simulink model "VFlexP"  (R2025a)
settings: Solver=ode23tb  StartTime=0.0  StopTime=40  FixedStep=5e-5
model workspace (MAT data in the model file):
  DCop_DCBUCK : object (value not decoded)
  Grid_CCVSC_idx = [2; 3; 4; 5; 6; 7; 8; 9; 10; 11; 12]
  Grid_CCVSCs = 1
  Grid_CCVSCs_buses = 1
  Grid_CCVSCs_toM = [0 1 0 0 0 0 0 0 0 0 0 0 ... (781 elements, 71x11)]
  Grid_C_Lines = [0.1 0.1 0.1 0.1]
  Grid_Cbuses = [0.05000002 0.10000002 0.10000002 0.10000002 0.05000002]
  Grid_DC : object (value not decoded)
  Grid_DCop_DCBUCK : object (value not decoded)
  Grid_DCop_DC_PES : object (value not decoded)
  Grid_DFIGs = 1
  Grid_DFIGs_buses = 1
  Grid_DGs : string (value not decoded)
  Grid_From_buses = [1 2 4 4]
  Grid_GFls = 1
  Grid_GFls_buses = 1
  Grid_GFr_idx = [1; 2; 3]
  Grid_GFrs = 1
  Grid_GFrs_buses = 1
  Grid_GFrs_toM = [1 0 0 0 0 0 0 0 0 1 0 0 ... (15 elements, 5x3)]
  Grid_IG_idx = 1
  Grid_IGs = 1
  Grid_IGs_buses = 1
  Grid_IGs_toM = [1; 0]
  Grid_L_Lines = [0.5 0.5 0.5 0.5]
  Grid_L_Loads = [0.000959999944704 0.000156249997559 0.00154855477548]
  Grid_Lines_fromM : object (value not decoded)
  Grid_Lines_toM : object (value not decoded)
  Grid_Load_buses = [2; 3; 4]
  Grid_Load_busesDC = []
  Grid_MGES_idx = [1; 2; 3]
  Grid_MGESs = 1
  Grid_MGESs_buses = [1; 5; 3]
  Grid_MGESs_toM = [1 0 0 0 0 0 0 0 0 1 0 0 ... (15 elements, 5x3)]
  Grid_MSGs = 1
  Grid_MSGs_buses = 1
  Grid_Nbuses = 5
  Grid_PQ_gen = [3; 2; 2]
  Grid_Ploads = [1250 4000 1250]
  Grid_PloadsDC = []
  Grid_Ps_lf = [0.274439537683 0.78 0.3]
  Grid_Qloads = [0.3 0.5 0.5]
  Grid_Qs_lf = [-0.0366071562958 0.126505596722 -0.0162964024532]
  Grid_R_Lines = [0.01 0.01 0.01 0.01]
  Grid_R_Loads = [3.9999997696 1.24999998047 3.8713869387]
  Grid_R_Loads_DC = 0
  Grid_Rcf = [50000000 50000000 50000000 50000000 50000000]
  Grid_SCs = 1
  Grid_SCs_buses = 1
  Grid_SG_idx = 1
  Grid_SGs = 1
  Grid_SGs_buses = 1
  Grid_SGs_toM = [1; 0]
  Grid_To_buses = [2 3 3 5]
  Grid_VCVSC_idx = [1; 2; 3; 4; 5; 6; 7; 8; 9; 10; 11; 12]
  Grid_VCVSCs = 1
  Grid_VCVSCs_buses = [1; 2; 3; 6; 8; 9; 12; 58; 59; 60; 63; 65]
  Grid_VCVSCs_toM = [1 0 0 0 0 0 0 0 0 0 0 0 ... (852 elements, 71x12)]
  Grid_VSM_idx = [1; 2; 3]
  Grid_VSMs = 1
  Grid_VSMs_buses = 1
  Grid_VSMs_toM = [1 0 0 0 0 0 0 0 0 1 0 0 ... (15 elements, 5x3)]
  Grid_admitt_matrix = [2.15353135314-19.7953135314i  -1.9801980198+19.801980198i; -1.9801980198+19.801980198i  2.15353135314-19.7953135314i]
  Grid_admitt_matrix_noloads = [1.98686468647-19.7953135314i  -1.9801980198+19.801980198i; -1.9801980198+19.801980198i  1.98686468647-19.7953135314i]
  Grid_bus = [1; 2; 6; 7; 8]
  Grid_busDC_complexity = [1 1 1]
  Grid_busDC_complexity_PF = [2 2 2]
  Grid_bus_complexity = [1 1 1 1 1]
  Grid_bus_complexity_PF = [1 1 1 1 1]
  Grid_buses_lf = [1; 5; 3]
  Grid_conductance_matrix = [100.00000002  -100  0; -100  200.00000002  -100; 0  -100  100.00000002]
  Grid_conductance_matrix_noloads = [100.00000002  -100  0; -100  200.00000002  -100; 0  -100  100.00000002]
  Grid_fref : object (value not decoded)
  Grid_gen_static_params : mBase (value not decoded)
  Grid_iPs_lf = [3.64378984326 1.28205128205 3.33333333333]
  Grid_iQs_lf = [-27.3170631425 7.90478860943 -61.3632366329]
  Grid_iadmitt_matrix = [2.88165849328-0.0982918688642i  2.87905051706-0.123273862303i; 2.87905051706-0.123273862303i  2.88165849328-0.0982918688642i]
  Grid_iadmitt_matrix_noloads = [37.5012524798-37.4874983544i  37.4987475202-37.5125016456i; 37.4987475202-37.5125016456i  37.5012524798-37.4874983544i]
  Grid_iconductance_matrix = [16666671.4556  16666671.4489  16666671.4456; 16666671.4489  16666671.4522  16666671.4489; 16666671.4456  16666671.4489  16666671.4556]
  Grid_iconductance_matrix_noloads = [16666671.4556  16666671.4489  16666671.4456; 16666671.4489  16666671.4522  16666671.4489; 16666671.4456  16666671.4489  16666671.4556]
  Grid_init_OK_bool = 1
  Grid_intconv_PF : object (value not decoded)
  Grid_lf_op : op_report (value not decoded)
  Grid_lineDC_complexity = [1 1]
  Grid_lineDC_complexity_PF = [2 2]
  Grid_line_complexity = [1 1 1 1]
  Grid_line_complexity_PF = [3 3 3 3]
  Grid_loadDC_complexity = []
  Grid_loadDC_complexity_PF = []
  Grid_load_complexity = [3 3 3]
  Grid_load_complexity_PF = [4 4 4]
  Grid_opDC_CCVSC : object (value not decoded)
  Grid_opDC_VSM : object (value not decoded)
  Grid_opGFr : object (value not decoded)
  Grid_opVCVSC : object (value not decoded)
  Grid_op_CCVSC : object (value not decoded)
  Grid_op_IG : object (value not decoded)
  Grid_op_MGES : object (value not decoded)
  Grid_op_SG : object (value not decoded)
  Grid_op_VSM : object (value not decoded)
  Grid_shift_lines = [0 0 0 0]
  Grid_tap_lines = [1 1 1 1]
  Grid_v_buses_mod = [1 1 1 0.9837920967 1]
  LinsysParamChangeStruct : Param1 (value not decoded)
  Lline = 0.01
  Rline = 1e-05
  linsys : object (value not decoded)
symbols that are objects in the model workspace (value not decoded): Grid_DCop_DC_PES, Grid_DCop_DCBUCK, Grid_op_CCVSC, Grid_op_IG, Grid_op_MGES, Grid_op_SG, Grid_op_VSM, Grid_opDC_CCVSC, Grid_opDC_VSM, Grid_opGFr, Grid_opVCVSC
undefined symbols (not defined in the file): block_buses_DC, block_idx, CCVSC_idx, Cf, costs, costs2, D, DFIGs_nodes, DiscIntNeverNeededParam, entity, Fb, Fi, From_nodes, grid_linsys, Grid_op_DFIG, Grid_op_DFIG_PQ, Grid_op_MSG, Grid_op_SC, Grid_op_VCVSC, H, initial_states_grid, K_1, K_3, K_5, K_A, K_C, K_IM, K_IR, K_P, K_PM, K_PR, K_S1, K_S2, K_S3, Ki_w, Kic, Kiv, Kp_id, Kp_theta, Kp_w, Kpc, Kpv, last_send, Lc, Lf, Lfd, Lkd1, Lkd2, Lkq1, Lkq2, Lkq3, Lmd, Lmq, Lsd, Lsq, m, M, Matrix_flux_to_i, mp, MSGs_buses ... (+44)
libraries: simulink x1048, eeGeneralControl x12
(part 27 of 50)

== system VFlexP/Grid/Generators/DFIG/GSC Control/PI Estator Current d ==
  in : Inport
  Gain : Gain  Gain=Kp_ia
  Gain1 : Gain  Gain=Ki_ia
  Sum : Sum  Inputs=++|
  xa2 : Integrator  InitialCondition=Grid_op_DFIG.op.States(4).x'
  out : Outport  VectorParamsAs1DForOutWhenUnconnected=off
  wires:
  xa2/1 -> Sum/2
  Gain/1 -> Sum/1
  in/1 -> Gain1/1, Gain/1
  Sum/1 -> out/1
  Gain1/1 -> xa2/1

== system VFlexP/Grid/Generators/DFIG/GSC Control/PI Estator Current q ==
  in : Inport
  Gain : Gain  Gain=Kp_ia
  Gain1 : Gain  Gain=Ki_ia
  Sum : Sum  Inputs=++|
  xa1 : Integrator  InitialCondition=Grid_op_DFIG.op.States(5).x'
  out : Outport  VectorParamsAs1DForOutWhenUnconnected=off
  wires:
  Gain1/1 -> xa1/1
  Sum/1 -> out/1
  in/1 -> Gain/1, Gain1/1
  Gain/1 -> Sum/1
  xa1/1 -> Sum/2

== system VFlexP/Grid/Generators/DFIG/GSC Control/Subsystem1 ==
  ws : Inport
  vaq' : Inport  Port=2
  vsq : Inport  Port=3
  iad : Inport  Port=4
  Gain1 : Gain  Gain=La_pu
  Product1 : Product
  Sum4 : Sum  Inputs=-|+|-  InputSameDT=on  SaturateOnIntegerOverflow=on  OutDataTypeStr=Inherit: Same as first input
  vadq : Outport
  wires:
  iad/1 -> Product1/2
  Gain1/1 -> Product1/1
  vaq'/1 -> Sum4/1
  Sum4/1 -> vadq/1  "vadq"
  Product1/1 -> Sum4/3
  ws/1 -> Gain1/1
  vsq/1 -> Sum4/2

== system VFlexP/Grid/Generators/DFIG/GSC Control/Subsystem3 ==
  vad' : Inport
  vd : Inport  Port=2
  iaq : Inport  Port=3
  ws : Inport  Port=4
  Gain1 : Gain  Gain=La_pu
  Product1 : Product
  Sum4 : Sum  Inputs=-|+|+  InputSameDT=on  SaturateOnIntegerOverflow=on  OutDataTypeStr=Inherit: Same as first input
  vad : Outport
  wires:
  iaq/1 -> Product1/2
  ws/1 -> Gain1/1
  Product1/1 -> Sum4/3
  Sum4/1 -> vad/1  "vadq"
  vd/1 -> Sum4/2
  vad'/1 -> Sum4/1
  Gain1/1 -> Product1/1

== system VFlexP/Grid/Generators/DFIG/RSC Control/PI Rotor Current d ==
  in : Inport
  Gain : Gain  Gain=Kp_ir
  Gain1 : Gain  Gain=Ki_ir
  Sum : Sum  Inputs=++|
  xr1 : Integrator  InitialCondition=Grid_op_DFIG.op.States(12).x'
  out : Outport  VectorParamsAs1DForOutWhenUnconnected=off
  wires:
  Gain1/1 -> xr1/1
  Sum/1 -> out/1
  in/1 -> Gain/1, Gain1/1
  Gain/1 -> Sum/1
  xr1/1 -> Sum/2

== system VFlexP/Grid/Generators/DFIG/RSC Control/PI Rotor Current q ==
  in : Inport
  Gain : Gain  Gain=Kp_ir
  Gain1 : Gain  Gain=Ki_ir
  Sum : Sum  Inputs=++|
  xr2 : Integrator  InitialCondition=Grid_op_DFIG.op.States(13).x'
  out : Outport  VectorParamsAs1DForOutWhenUnconnected=off
  wires:
  xr2/1 -> Sum/2
  Gain/1 -> Sum/1
  in/1 -> Gain1/1, Gain/1
  Sum/1 -> out/1
  Gain1/1 -> xr2/1

== system VFlexP/Grid/Generators/DFIG/Slip/PI Slip ==
  in : Inport
  Gain : Gain  Gain=Kp_s
  Gain1 : Gain  Gain=Ki_s
  Sum : Sum  Inputs=++|
  xr3 : Integrator  InitialCondition=Grid_op_DFIG_PQ.op.States(16).x'  UpperSaturationLimit=1.01  LowerSaturationLimit=0.99
  out : Outport  VectorParamsAs1DForOutWhenUnconnected=off
  wires:
  xr3/1 -> Sum/2
  Gain/1 -> Sum/1
  in/1 -> Gain1/1, Gain/1
  Sum/1 -> out/1
  Gain1/1 -> xr3/1

== system VFlexP/Grid/Generators/DFIG/Stator circuit/Subsystem1 ==
  vd : Inport
  vq : Inport  Port=2
  id : Inport  Port=3
  iq : Inport  Port=4
  s*ws : Inport  Port=5
  Gain1 : Gain  Gain=Rr_pu
  Gain6 : Gain  Gain=Rr_pu
  Gain7 : Gain  Gain=-1
  Product{1..4} (4 alike) : Product
  Selector8 : Selector  InputPortWidth=length(fref.ref_units)  IndexOptions=Index vector (dialog)  Indices=block_fref  OutputSizes=1
  Sum1 : Sum  Inputs=-|+|-  InputSameDT=on  SaturateOnIntegerOverflow=on  OutDataTypeStr=Inherit: Same as first input
  Sum4 : Sum  Inputs=-|+|-  InputSameDT=on  SaturateOnIntegerOverflow=on  OutDataTypeStr=Inherit: Same as first input
  psis_d : Integrator  InitialCondition=Grid_op_DFIG.op.States(15).x'
  psis_q : Integrator  InitialCondition=Grid_op_DFIG.op.States(16).x'
  d : Outport
  q : Outport  Port=2
  wires:
  Product1/1 -> Sum4/1
  s*ws/1 -> Product1/1, Product2/2
  Gain6/1 -> Sum4/3
  Product3/1 -> psis_q/1
  Sum1/1 -> Product4/1
  psis_d/1 -> Product1/2, d/1
  Sum4/1 -> Product3/2
  Product4/1 -> psis_d/1
  Gain1/1 -> Sum1/1
  Gain7/1 -> Product2/1
  id/1 -> Gain1/1
  Product2/1 -> Sum1/3
  psis_q/1 -> q/1, Gain7/1
  iq/1 -> Gain6/1
  vd/1 -> Sum1/2
  vq/1 -> Sum4/2
  Selector8/1 -> Product3/1, Product4/2
  [omega_base] -> Selector8/1

== system VFlexP/Grid/Generators/DFIG/Stator circuit/Subsystem2 ==
  vad : Inport
  vaq : Inport  Port=2
  id : Inport  Port=3
  iq : Inport  Port=4
  ws : Inport  Port=5
  vsd : Inport  Port=6
  vsq : Inport  Port=7
  Gain1 : Gain  Gain=Ra_pu
  Gain6 : Gain  Gain=Ra_pu
  Gain7 : Gain  Gain=-1
  Product{1..4} (4 alike) : Product
  Selector8 : Selector  InputPortWidth=length(fref.ref_units)  IndexOptions=Index vector (dialog)  Indices=block_fref  OutputSizes=1
  Sum1 : Sum  Inputs=-|+|-|-  InputSameDT=on  SaturateOnIntegerOverflow=on  OutDataTypeStr=Inherit: Same as first input
  Sum2 : Sum  Inputs=-|+|-|-  InputSameDT=on  SaturateOnIntegerOverflow=on  OutDataTypeStr=Inherit: Same as first input
  psis_d : Integrator  InitialCondition=Grid_op_DFIG.op.States(17).x'
  psis_q : Integrator  InitialCondition=Grid_op_DFIG.op.States(18).x'
  d : Outport
  q : Outport  Port=2
  wires:
  iq/1 -> Gain6/1
  psis_q/1 -> Gain7/1, q/1
  Product2/1 -> Sum1/3
  id/1 -> Gain1/1
  Gain7/1 -> Product2/1
  Gain1/1 -> Sum1/1
  Product4/1 -> psis_d/1
  Sum2/1 -> Product3/2
  psis_d/1 -> Product1/2, d/1
  Sum1/1 -> Product4/1
  Product3/1 -> psis_q/1
  ws/1 -> Product2/2, Product1/1
  vsd/1 -> Sum1/2
  vad/1 -> Sum1/4
  Gain6/1 -> Sum2/4
  vsq/1 -> Sum2/2
  Product1/1 -> Sum2/1
  vaq/1 -> Sum2/3
  Selector8/1 -> Product3/1, Product4/2
  [omega_base] -> Selector8/1

== system VFlexP/Grid/Generators/DFIG/Stator circuit/Subsystem3 ==
  vd : Inport
  vq : Inport  Port=2
  id : Inport  Port=3
  iq : Inport  Port=4
  ws : Inport  Port=5
  Gain1 : Gain  Gain=Rs_pu
  Gain6 : Gain  Gain=Rs_pu
  Gain7 : Gain  Gain=-1
  Product{1..4} (4 alike) : Product
  Selector8 : Selector  InputPortWidth=length(fref.ref_units)  IndexOptions=Index vector (dialog)  Indices=block_fref  OutputSizes=1
  Sum1 : Sum  Inputs=-|+|-  InputSameDT=on  SaturateOnIntegerOverflow=on  OutDataTypeStr=Inherit: Same as first input
  Sum4 : Sum  Inputs=-|+|-  InputSameDT=on  SaturateOnIntegerOverflow=on  OutDataTypeStr=Inherit: Same as first input
  psis_d : Integrator  InitialCondition=Grid_op_DFIG.op.States(19).x'
  psis_q : Integrator  InitialCondition=Grid_op_DFIG.op.States(20).x'
  d : Outport
  q : Outport  Port=2
  wires:
  vq/1 -> Sum4/2
  vd/1 -> Sum1/2
  iq/1 -> Gain6/1
  psis_q/1 -> q/1, Gain7/1
  Product2/1 -> Sum1/3
  id/1 -> Gain1/1
  Gain7/1 -> Product2/1
  Product4/1 -> psis_d/1
  Sum4/1 -> Product3/2
  psis_d/1 -> d/1, Product1/2
  Sum1/1 -> Product4/1
  Product3/1 -> psis_q/1
  ws/1 -> Product2/2, Product1/1
  Product1/1 -> Sum4/1
  Gain1/1 -> Sum1/1
  Gain6/1 -> Sum4/3
  Selector8/1 -> Product3/1, Product4/2
  [omega_base] -> Selector8/1

== system VFlexP/Grid/Generators/DFIG/Vc control/PI Vc2 ==
  in : Inport
  Gain : Gain  Gain=Kp_vc2
  Gain1 : Gain  Gain=Ki_vc2
  Sum : Sum  Inputs=++|
  xa3 : Integrator  InitialCondition=Grid_op_DFIG.op.States(22).x'
  out : Outport  VectorParamsAs1DForOutWhenUnconnected=off
  wires:
  Gain1/1 -> xa3/1
  Sum/1 -> out/1
  in/1 -> Gain/1, Gain1/1
  Gain/1 -> Sum/1
  xa3/1 -> Sum/2

== system VFlexP/Grid/Generators/GFl/CC/dynamic ==
  idref : Inport
  iqref : Inport  Port=2
  vod : Inport  Port=3
  voq : Inport  Port=4
  omega : Inport  Port=5
  "Lf " : Gain  Gain=Lf
  Lf1 : Gain  Gain=Lf
  Product : Product
  Product3 : Product
  RL : Subsystem  Variant=on  VariantControlMode=label  LabelModeActiveChoice=dynamic  mask(Line){dynamic=Dynamic, R=Rf, L=Lf}
      mask prompts: dynamic "Dynamic behavior"; R "Series resistance (p.u.)"; L "Inductance (p.u.)"
      mask init: same as VFlexP/Grid/Generators/GFr/RL out
      mask Help: web('Documentation/RL.html')
      mask TypeOptions dynamic: Static | Dynamic | Static omega
  Subsystem : Subsystem
  Subsystem1 : Subsystem
  Sum1 : Sum  Inputs=++|
  Sum2 : Sum  Inputs=++|
  Sum8 : Sum  Inputs=-+|
  Sum9 : Sum  Inputs=|++
  idiref : Outport
  iqiref : Outport  Port=2
  wires:
  RL/2(iq) -> iqiref/1, Subsystem1/2(y), "Lf "/1
  Subsystem1/1(Out1) -> Sum9/1
  [omega] -> Product3/1  "omega"
  "Lf "/1 -> Product/1
  Product3/1 -> Sum9/2
  Lf1/1 -> Product3/2
  [omega] -> Product/2
  Product/1 -> Sum8/1
  iqref/1 -> Subsystem1/1(ref)  "iqref"
  Sum8/1 -> Sum1/2
  Sum9/1 -> Sum2/2
  [vod] -> Sum1/1
  [voq] -> Sum2/1
  omega/1 -> [omega]  "omega"
  voq/1 -> [voq]  "ioq"
  vod/1 -> [vod]  "iod"
  [vod] -> RL/2(v_out_d)
  [voq] -> RL/4(v_out_q)
  Sum1/1 -> RL/1(v_in_d)
  Sum2/1 -> RL/3(v_in_q)
  RL/1(id) -> Subsystem/2(y), Lf1/1, idiref/1
  idref/1 -> Subsystem/1(ref)  "idref"
  Subsystem/1(Out1) -> Sum8/2
  [omega] -> RL/5(omega)

== system VFlexP/Grid/Generators/GFl/CC/static ==
  idref : Inport
  iqref : Inport  Port=2
  vod : Inport  Port=3
  voq : Inport  Port=4
  omega : Inport  Port=5
  Terminator : Terminator
  Terminator1 : Terminator
  Terminator2 : Terminator
  idiref : Outport
  iqiref : Outport  Port=2
  wires:
  voq/1 -> Terminator1/1  "voq"
  vod/1 -> Terminator/1  "vod"
  idref/1 -> idiref/1  "idref"
  iqref/1 -> iqiref/1  "iqref"
  omega/1 -> Terminator2/1  "omega"

== system VFlexP/Grid/Generators/GFl/PC/LPF_d ==
  In1 : Inport
  Gain : Gain  Gain=iTf
  I : Integrator  InitialCondition=Grid_op_CCVSC.op.States(8).x'
  Sum4 : Sum  Inputs=|+-
  Out1 : Outport
  wires:
  Gain/1 -> I/1
  Sum4/1 -> Gain/1
  In1/1 -> Sum4/1
  I/1 -> Sum4/2, Out1/1

== system VFlexP/Grid/Generators/GFl/PC/LPF_q ==
  In1 : Inport
  Gain : Gain  Gain=iTf
  I : Integrator  InitialCondition=Grid_op_CCVSC.op.States(9).x'
  Sum4 : Sum  Inputs=|+-
  Out1 : Outport
  wires:
  Gain/1 -> I/1
  I/1 -> Sum4/2, Out1/1
  In1/1 -> Sum4/1
  Sum4/1 -> Gain/1

== system VFlexP/Grid/Generators/GFl/PC/Saturation ==
  ildref : Inport
  ilqref : Inport  Port=2
  Abs : Abs  ZeroCross=off  SaturateOnIntegerOverflow=off
  Abs1 : Abs  ZeroCross=off  SaturateOnIntegerOverflow=off
  Abs2 : Abs  ZeroCross=off  SaturateOnIntegerOverflow=off
  Divide2 : Product  Inputs=*/
  Divide3 : Product  Inputs=*/
  Gain : Gain  Gain=-1
  Gain3 : Gain  Gain=-1
  Real-Imag to Complex : RealImagToComplex
  Saturation Dynamic : simulink/Discontinuities/Saturation Dynamic  OutMin=[]  OutMax=[]  OutDataTypeStr=Inherit: Same as second input  OutDataType=fixdt(1, 16)  OutScaling=2^-10  DoSatur=off
  Saturation Dynamic1 : simulink/Discontinuities/Saturation Dynamic  OutMin=[]  OutMax=[]  OutDataTypeStr=Inherit: Same as second input  OutDataType=fixdt(1, 16)  OutScaling=2^-10  DoSatur=off
  y : Outport
  y1 : Outport  Port=2
  wires:
  Gain/1 -> Saturation Dynamic1/3
  Divide3/1 -> Gain/1, Saturation Dynamic1/1
  Divide2/1 -> Gain3/1, Saturation Dynamic/1
  Saturation Dynamic/1 -> y/1
  Abs/1 -> Divide3/2, Divide2/2
  Gain3/1 -> Saturation Dynamic/3
  Abs1/1 -> Divide3/1
  Real-Imag to Complex/1 -> Abs/1
  ilqref/1 -> Abs1/1, Saturation Dynamic1/2, Real-Imag to Complex/2
  Abs2/1 -> Divide2/1
  ildref/1 -> Abs2/1, Saturation Dynamic/2, Real-Imag to Complex/1
  Saturation Dynamic1/1 -> y1/1

== system VFlexP/Grid/Generators/GFl/PLL/dynamic ==
  vq : Inport
  omega : Inport  Port=2
  voutangle : Inport  Port=3
  PLL : Subsystem
  Product : Product
  Selector8 : Selector  InputPortWidth=length(fref.ref_units)  IndexOptions=Index vector (dialog)  Indices=block_fref  OutputSizes=1
  Sum2 : Sum  Inputs=|-+
  Sum3 : Sum  Inputs=+-|
  Terminator : Terminator
  Zero : Constant  Value=0  OutDataTypeStr=Inherit: Inherit via back propagation
  frame : Integrator  InitialCondition=Grid_op_CCVSC.op.States(7).x'  UpperSaturationLimit=pi  LowerSaturationLimit=-pi
  theta : Outport
  omega_point : Outport  Port=2
  wires:
  voutangle/1 -> Terminator/1
  vq/1 -> Sum2/2  "vq"
  omega/1 -> Sum3/2  "omega"
  Zero/1 -> Sum2/1
  frame/1 -> theta/1  "theta"
  Product/1 -> frame/1
  PLL/1(Input2) -> omega_point/1, Sum3/1  "omega2"
  Sum3/1 -> Product/1
  Sum2/1 -> PLL/1(In1)
  [omega_base] -> Selector8/1
  Selector8/1 -> Product/2

== system VFlexP/Grid/Generators/GFl/PLL/static ==
  vq : Inport
  omega : Inport  Port=2
  voutangle : Inport  Port=3
  Gain : Gain  Gain=-1
  Terminator : Terminator
  Terminator1 : Terminator
  Transport Delay : TransportDelay  DelayTime=1e-6  TransDelayFeedthrough=on
  theta : Outport
  omega_point : Outport  Port=2
  wires:
  Transport Delay/1 -> theta/1
  Gain/1 -> Transport Delay/1
  vq/1 -> Terminator/1  "vq"
  omega/1 -> omega_point/1, Terminator1/1  "vq"
  voutangle/1 -> Gain/1

== system VFlexP/Grid/Generators/GFr/PC/LPF_P ==
  P : Inport
  Gain : Gain  Gain=iTf
  I : Integrator
  Sum4 : Sum  Inputs=|+-
  P_f : Outport
  wires:
  Gain/1 -> I/1
  Sum4/1 -> Gain/1
  P/1 -> Sum4/1
  I/1 -> P_f/1, Sum4/2

== system VFlexP/Grid/Generators/GFr/PC/LPF_Q ==
  Q : Inport
  Gain : Gain  Gain=iTf
  I : Integrator
  Sum4 : Sum  Inputs=|+-
  Q_f : Outport
  wires:
  Gain/1 -> I/1
  Q/1 -> Sum4/1
  I/1 -> Q_f/1, Sum4/2
  Sum4/1 -> Gain/1

== system VFlexP/Grid/Generators/GFr/RL out/dynamic ==
  v_in_d : Inport
  v_out_d : Inport  Port=2
  v_in_q : Inport  Port=3
  v_out_q : Inport  Port=4
  Gain1 : Gain  Gain=L
  Gain2 : Gain  Gain=R
  Gain3 : Gain  Gain=R
  Gain4 : Gain  Gain=L
  Gain5 : Gain  Gain=invL
  Gain7 : Gain  Gain=invL
  Product{,1..3} (4 alike) : Product
  Selector1 : Selector  InputPortWidth=length(fref.ref_units)  IndexOptions=Index vector (dialog)  Indices=block_fref  OutputSizes=1
  Selector7 : Selector  InputPortWidth=length(fref.ref_units)  IndexOptions=Index vector (dialog)  Indices=block_fref  OutputSizes=1
  Sum4 : Sum  Inputs=+-|
  Sum5 : Sum  Inputs=|-+
  Sum6 : Sum  Inputs=|++
  Sum7 : Sum  Inputs=-+|
  Sum8 : Sum  Inputs=|+-
  Sum9 : Sum  Inputs=-+|
  i_d : Integrator  InitialCondition=Grid_opGFr.id_out
  i_q : Integrator  InitialCondition=Grid_opGFr.iq_out
  id : Outport
  iq : Outport  Port=2
  v_outd : Outport  Port=3
  v_outq : Outport  Port=4
  wires:
  v_out_q/1 -> v_outq/1, Sum9/1  "v_out_q"
  v_out_d/1 -> v_outd/1, Sum7/1  "v_out_d"
  Sum9/1 -> Sum8/1
  Gain1/1 -> Product1/2
  i_q/1 -> iq/1, Gain4/1, Gain3/1  "iq"
  Sum5/1 -> Sum9/2
  Gain3/1 -> Sum5/1
  Sum7/1 -> Sum6/1
  Gain4/1 -> Product/1
  Product1/1 -> Sum8/2
  Sum4/1 -> Sum7/2
  Sum8/1 -> Gain7/1
  Product/1 -> Sum6/2
  [omega_ref] -> Selector7/1  "omega"
  Sum6/1 -> Gain5/1
  i_d/1 -> id/1, Gain1/1, Gain2/1  "id"
  Gain2/1 -> Sum4/2
  v_in_d/1 -> Sum4/1  "v_in_d"
  v_in_q/1 -> Sum5/2  "v_in_q"
  Selector7/1 -> Product/2, Product1/1
  Selector1/1 -> Product2/2, Product3/1
  [omega_base] -> Selector1/1
  Product3/1 -> i_q/1
  Gain7/1 -> Product3/2
  Gain5/1 -> Product2/1
  Product2/1 -> i_d/1

== system VFlexP/Grid/Generators/GFr/RL out/static ==
  v_in_d : Inport
  v_out_d : Inport  Port=2
  v_in_q : Inport  Port=3
  v_out_q : Inport  Port=4
  Constant : Constant  Value=R.^2
  Constant1 : Constant
  Divide : Product  Inputs=*/
  Gain : Gain  Gain=L
  Gain1 : Gain  Gain=R
  Gain2 : Gain  Gain=R
  Product{,1..5} (6 alike) : Product
  Selector7 : Selector  InputPortWidth=length(fref.ref_units)  IndexOptions=Index vector (dialog)  Indices=block_fref  OutputSizes=1
  Sum : Sum  Inputs=|++
  Sum1 : Sum  Inputs=|+-
  Sum2 : Sum  Inputs=|+-
  Sum3 : Sum  Inputs=|++
  Sum4 : Sum  Inputs=|-+
  id : Outport
  iq : Outport  Port=2
  v_outd : Outport  Port=3
  v_outq : Outport  Port=4
  wires:
  v_in_d/1 -> Sum1/1  "v_in_d"
  v_out_q/1 -> v_outq/1, Sum2/2  "v_out_q"
  Sum4/1 -> iq/1  "iq"
  Sum3/1 -> id/1  "id"
  Gain1/1 -> Product1/2
  Product2/1 -> Product4/2, Product3/1
  Product4/1 -> Sum4/1
  Divide/1 -> Gain2/1, Gain1/1, Product2/1
  Sum1/1 -> Product1/1, Product4/1  "vd"
  Product3/1 -> Sum3/2
  Constant1/1 -> Divide/1
  Gain/1 -> Product/2, Product/1, Product2/2
  Sum2/1 -> Product5/1, Product3/2  "vq"
  Constant/1 -> Sum/1
  Product5/1 -> Sum4/2
  Product1/1 -> Sum3/1
  Product/1 -> Sum/2
  Gain2/1 -> Product5/2
  Sum/1 -> Divide/2
  v_out_d/1 -> v_outd/1, Sum1/2  "v_out_d"
  v_in_q/1 -> Sum2/1  "v_in_q"
  [omega_ref] -> Selector7/1  "omega"
  Selector7/1 -> Gain/1

== system VFlexP/Grid/Generators/GFr/RL out/static_omega ==
  v_in_d : Inport
  v_out_d : Inport  Port=2
  v_in_q : Inport  Port=3
  v_out_q : Inport  Port=4
  Gain : Gain  Gain=1./(R.^2+L.^2)
  Gain2 : Gain  Gain=1./(R.^2+L.^2)
  Gain3 : Gain  Gain=R
  Gain4 : Gain  Gain=L
  Gain5 : Gain  Gain=L
  Gain6 : Gain  Gain=R
  Sum : Sum  Inputs=|++
  Sum1 : Sum  Inputs=|+-
  Sum2 : Sum  Inputs=|+-
  Sum3 : Sum  Inputs=|-+
  id : Outport
  iq : Outport  Port=2
  v_outd : Outport  Port=3
  v_outq : Outport  Port=4
  wires:
  v_in_q/1 -> Sum2/1  "v_in_q"
  v_in_d/1 -> Sum1/1  "v_in_d"
  v_out_q/1 -> v_outq/1, Sum2/2  "v_out_q"
  v_out_d/1 -> v_outd/1, Sum1/2  "v_out_d"
  Sum1/1 -> Gain/1  "vd"
  Sum2/1 -> Gain2/1  "vq"
  Gain/1 -> Gain5/1, Gain3/1
  Gain3/1 -> Sum/1
  Gain4/1 -> Sum/2
  Gain2/1 -> Gain6/1, Gain4/1
  Sum/1 -> id/1
  Gain5/1 -> Sum3/1
  Sum3/1 -> iq/1
  Gain6/1 -> Sum3/2

== system VFlexP/Grid/Generators/GFr/VCC/dynamic ==
  vodref : Inport
  voqref : Inport  Port=2
  iod : Inport  Port=3
  ioq : Inport  Port=4
  omega : Inport  Port=5
  Cf : Gain  Gain=Cfi
  Cf 1 : Gain  Gain=Cfi
  Constant : Constant  Value=Tint==Inf  VectorParams1D=off
  Constant1 : Constant  Value=Text==Inf  VectorParams1D=off
  Fi : Gain  Gain=Fi
  Fi2 : Gain  Gain=Fi
  "Lf " : Gain  Gain=Lf
  Lf1 : Gain  Gain=Lf
  PIid : Subsystem
  PIiq : Subsystem
  PIvd : Subsystem
  PIvq : Subsystem
  Product{,1..3} (4 alike) : Product
  RC : Subsystem  Variant=on  VariantControlMode=label  LabelModeActiveChoice=dynamic  mask{dynamic=Dynamic, R=Rcf, C=Cfi}
      mask prompts: dynamic "Dynamic behavior"; R "Parallel resistance (p.u.)"; C "Capacitance (p.u.)"
      mask init: same as VFlexP/Grid/DCAC converters/DC_VSM/VCC/dynamic_limiting/RC
      mask TypeOptions dynamic: Dynamic | Static | Static omega
  RL : Subsystem  Variant=on  VariantControlMode=label  LabelModeActiveChoice=dynamic  mask(Line){dynamic=Dynamic, R=Rf, L=Lf}
      mask prompts: dynamic "Dynamic behavior"; R "Series resistance (p.u.)"; L "Inductance (p.u.)"
      mask init: same as VFlexP/Grid/Generators/GFr/RL out
      mask Help: web('Documentation/RL.html')
      mask TypeOptions dynamic: Static | Dynamic | Static omega
  Subsystem : Subsystem
  Subsystem1 : Subsystem
  Sum1 : Sum  Inputs=++|
  Sum2 : Sum  Inputs=-+|
  Sum{3,5..6,9} (4 alike) : Sum  Inputs=|++
  Sum4 : Sum  Inputs=++|
  Sum8 : Sum  Inputs=-+|
  Switch{,1..3} (4 alike) : Switch  Criteria=u2 > Threshold  SaturateOnIntegerOverflow=off  InputSameDT=off
  vidref : Outport
  viqref : Outport  Port=2
  wires:
  Sum5/1 -> Switch1/1, PIiq/1(ref)  "ilqref"
  Product/1 -> Sum8/1
  vodref/1 -> Switch2/1, PIvd/1(ref)  "vodref"
  RC/2(vq) -> PIvq/2(y), Cf/1, Subsystem/4(In4), Sum6/2, Switch3/3  "voq"
  [omega] -> Product/2
  Lf1/1 -> Product3/2
  Fi/1 -> Sum4/1
  voqref/1 -> Switch3/1, PIvq/1(ref)  "voqref"
  Product3/1 -> Sum9/2
  Product2/1 -> Sum3/2
  Cf 1/1 -> Product2/2
  Cf/1 -> Product1/2
  Sum4/1 -> PIid/1(ref), Switch/1  "ildref"
  Product1/1 -> Sum2/1
  iod/1 -> Subsystem1/2(iod), Fi/1  "iod"
  Sum2/1 -> Sum4/2
  "Lf "/1 -> Product/1
  Sum3/1 -> Sum5/1
  [omega] -> Subsystem1/5(In5), Subsystem/5(In5), Product3/1  "omega"
  ioq/1 -> Subsystem1/4(ioq), Fi2/1  "ioq"
  Fi2/1 -> Sum5/2
  PIvd/1(Out1) -> Sum2/2
  PIvq/1(Out1) -> Sum3/1
  PIid/1(Out1) -> Sum8/2
  PIiq/1(Out1) -> Sum9/1
  omega/1 -> Product2/1, [omega]  "omega"
  [omega] -> Product1/1
  RC/1(vd) -> Subsystem/2(In2), Sum1/1, Switch2/3, PIvd/2(y), Cf 1/1
  RL/1(id) -> Switch/3, Lf1/1, PIid/2(y)
  RL/2(iq) -> Switch1/3, PIiq/2(y), "Lf "/1
  Sum8/1 -> Sum1/2  "vidref"
  Sum9/1 -> Sum6/1  "viqref"
  Sum1/1 -> Subsystem/1(In1)
  Sum6/1 -> Subsystem/3(In3)
  Subsystem/1(Out1) -> RL/1(v_in_d)
  Subsystem/2(Out2) -> RL/2(v_out_d)
  Subsystem/3(Out3) -> RL/3(v_in_q)
  Subsystem/4(Out4) -> RL/4(v_out_q)
  Subsystem/5(Out5) -> RL/5(omega)
  Subsystem1/1(Out1) -> RC/1(i_d_in)
  Subsystem1/2(Out2) -> RC/2(i_d_out)
  Subsystem1/3(Out3) -> RC/3(i_q_in)
  Subsystem1/4(Out4) -> RC/4(i_q_out)
  Subsystem1/5(Out5) -> RC/5(omega)
  Switch/1 -> Subsystem1/1(id)
  Switch1/1 -> Subsystem1/3(iq)
  Constant/1 -> Switch1/2, Switch/2
  Switch2/1 -> vidref/1
  Constant1/1 -> Switch3/2, Switch2/2
  Switch3/1 -> viqref/1

== system VFlexP/Grid/Generators/GFr/VCC/dynamic_VC ==
  vodref : Inport
  voqref : Inport  Port=2
  iod : Inport  Port=3
  ioq : Inport  Port=4
  omega : Inport  Port=5
  Cf : Gain  Gain=Cfi
  Cf 1 : Gain  Gain=Cfi
  Fi : Gain  Gain=Fi
  Fi2 : Gain  Gain=Fi
  Product1 : Product
  Product2 : Product
  RC : Subsystem  Variant=on  VariantControlMode=label  LabelModeActiveChoice=dynamic  mask{dynamic=Dynamic, R=Rcf, C=Cfi}
      mask prompts: dynamic "Dynamic behavior"; R "Parallel resistance (p.u.)"; C "Capacitance (p.u.)"
      mask init: same as VFlexP/Grid/DCAC converters/DC_VSM/VCC/dynamic_limiting/RC
      mask TypeOptions dynamic: Dynamic | Static | Static omega
  Subsystem : Subsystem
  Subsystem1 : Subsystem
  Sum2 : Sum  Inputs=-+|
  Sum3 : Sum  Inputs=|++
  Sum4 : Sum  Inputs=++|
  Sum5 : Sum  Inputs=|++
  vidref : Outport
  viqref : Outport  Port=2
  wires:
  [omega] -> Product1/1
  omega/1 -> RC/5(omega), Product2/1, [omega]  "omega"
  Subsystem1/1(Out1) -> Sum3/1
  Subsystem/1(Out1) -> Sum2/2
  Fi2/1 -> Sum5/2
  ioq/1 -> RC/4(i_q_out), Fi2/1  "ioq"
  Sum3/1 -> Sum5/1
  Sum2/1 -> Sum4/2
  iod/1 -> RC/2(i_d_out), Fi/1  "iod"
  Product1/1 -> Sum2/1
  Cf/1 -> Product1/2
  Cf 1/1 -> Product2/2
  Product2/1 -> Sum3/2
  voqref/1 -> Subsystem1/1(ref)  "voqref"
  Fi/1 -> Sum4/1
  RC/2(vq) -> viqref/1, Cf/1, Subsystem1/2(y)
  vodref/1 -> Subsystem/1(ref)  "vodref"
  RC/1(vd) -> vidref/1, Cf 1/1, Subsystem/2(y)
  Sum4/1 -> RC/1(i_d_in)
  Sum5/1 -> RC/3(i_q_in)

== system VFlexP/Grid/Generators/GFr/VCC/dynamic_limiting ==
  vodref : Inport
  voqref : Inport  Port=2
  iod : Inport  Port=3
  ioq : Inport  Port=4
  omega : Inport  Port=5
  Cf : Gain  Gain=Cfi
  Cf 1 : Gain  Gain=Cfi
  Complex to Magnitude-Angle2 : ComplexToMagnitudeAngle  Output=Magnitude
  Complex to Magnitude-Angle3 : ComplexToMagnitudeAngle
  Complex to Magnitude-Angle4 : ComplexToMagnitudeAngle  Output=Magnitude
  Complex to Magnitude-Angle5 : ComplexToMagnitudeAngle  Output=Magnitude
  Complex to Real-Imag1 : ComplexToRealImag
  Fi : Gain  Gain=Fi
  Fi2 : Gain  Gain=Fi
  "Lf " : Gain  Gain=Lf
  Lf1 : Gain  Gain=Lf
  Magnitude-Angle to Complex : MagnitudeAngleToComplex
  Memory : Memory
  NOT : Logic  Operator=NOT  IconShape=distinctive  AllPortsSameDT=off  OutDataTypeStr=boolean
  PIid : Subsystem
  PIiq : Subsystem
  PIvd : Subsystem
      settings: PortSchema="{\"entries\":[{\"content\":{\"sides\":[{\"content\":{\"connectorIds\":[\"In1\",\"In2\"]},\"type\":\"ConnectorPlacement.EquallySpacedRectSide\",\"uuid\":\"218efe14-094c-4cdd-8e62-ef6089c75bbd\"},{\"content\":{\"connectorIds\":[\"Out1\"],\"side\":\"RIGHT\"},\"type\":\"ConnectorPlacement.EquallySpacedRectSide\",\"uuid\":\"287e2a8a-062a-4519-a86c-f141c6982dac\"},{\"content\":{\"connectorIds\":[\"In3\"],\"side\":\"TOP\"},\"type\":\"ConnectorPlacement.EquallySpacedRectSide\",\"uuid\":\"e88fce21-908c-492a-b265-04b05ce94be8\"}]},\"type\":\"ConnectorPlacement.EquallySpacedConnector\",\"uuid\":\"5c149457-da6d-4223-b1cb-56365173b759\"}],\"packageUris\":[\"http://schema.mathworks.com/mf0/Connector/R2020b\"],\"version\":\"1.0\"}"
  PIvq : Subsystem
      settings: PortSchema="{\"entries\":[{\"content\":{\"sides\":[{\"content\":{\"connectorIds\":[\"In1\",\"In2\"]},\"type\":\"ConnectorPlacement.EquallySpacedRectSide\",\"uuid\":\"218efe14-094c-4cdd-8e62-ef6089c75bbd\"},{\"content\":{\"connectorIds\":[\"Out1\"],\"side\":\"RIGHT\"},\"type\":\"ConnectorPlacement.EquallySpacedRectSide\",\"uuid\":\"287e2a8a-062a-4519-a86c-f141c6982dac\"},{\"content\":{\"connectorIds\":[],\"side\":\"TOP\"},\"type\":\"ConnectorPlacement.EquallySpacedRectSide\",\"uuid\":\"e88fce21-908c-492a-b265-04b05ce94be8\"},{\"content\":{\"connectorIds\":[\"In3\"],\"side\":\"BOTTOM\"},\"type\":\"ConnectorPlacement.EquallySpacedRectSide\",\"uuid\":\"db964aea-37c6-4226-90b6-d177a6d2ab38\"}]},\"type\":\"ConnectorPlacement.EquallySpacedConnector\",\"uuid\":\"5c149457-da6d-4223-b1cb-56365173b759\"}],\"packageUris\":[\"http://schema.mathworks.com/mf0/Connector/R2020b\"],\"version\":\"1.0\"}"
  Product{,1..5} (6 alike) : Product
  RC : Subsystem  Variant=on  VariantControlMode=label  LabelModeActiveChoice=dynamic  mask{dynamic=Dynamic, R=Rcf, C=Cfi}
      mask prompts: dynamic "Dynamic behavior"; R "Parallel resistance (p.u.)"; C "Capacitance (p.u.)"
      mask init: same as VFlexP/Grid/DCAC converters/DC_VSM/VCC/dynamic_limiting/RC
      mask TypeOptions dynamic: Dynamic | Static | Static omega
  RL : Subsystem  Variant=on  VariantControlMode=label  LabelModeActiveChoice=dynamic  mask(Line){dynamic=Dynamic, R=Rf, L=Lf}
      mask prompts: dynamic "Dynamic behavior"; R "Series resistance (p.u.)"; L "Inductance (p.u.)"
      mask init: same as VFlexP/Grid/Generators/GFr/RL out
      mask Help: web('Documentation/RL.html')
      mask TypeOptions dynamic: Static | Dynamic | Static omega
  Real-Imag to Complex{2..5} (4 alike) : RealImagToComplex
  Relational Operator : RelationalOperator  Operator===  OutDataTypeStr=boolean  RndMeth=Simplest  InputSameDT=off
  Saturation : Saturate  UpperLimit=0.1  LowerLimit=0
  Scope{1,3,6..8} (5 alike) : Scope
      Scope1 settings: ActiveDisplayYMinimum=-0.06728  ActiveDisplayYMaximum=0.79818  DataLoggingVariableName=ScopeData2
      Scope3 settings: ActiveDisplayYMinimum=0.01769  ActiveDisplayYMaximum=0.10915
      Scope6 settings: ActiveDisplayYMinimum=0.03196  ActiveDisplayYMaximum=0.13112  DataLoggingVariableName=ScopeData2
      Scope7 settings: ActiveDisplayYMinimum=0.86043  ActiveDisplayYMaximum=1.1554  DataLoggingVariableName=ScopeData3
      Scope8 settings: ActiveDisplayYMinimum=0.0318  ActiveDisplayYMaximum=0.12782  DataLoggingVariableName=ScopeData4
  Scope2 : Scope  NumInputPorts=2
      settings: ActiveDisplayYMinimum=-0.10019  ActiveDisplayYMaximum=0.20176
  Scope4 : Scope  NumInputPorts=2
      settings: ActiveDisplayYMinimum=-0.04364  ActiveDisplayYMaximum=0.0791  DataLoggingVariableName=ScopeData3
  Sum1 : Sum  Inputs=++|
  Sum{3,5..6,9,14..15} (6 alike) : Sum  Inputs=|++
  Sum2 : Sum  Inputs=-+|
  Sum4 : Sum  Inputs=++|
  Sum8 : Sum  Inputs=-+|
  VI : Subsystem  mask{L=0.5, R=0.1, Tf=0}
      mask prompts: L "Inductance (pu)"; R "Resistance (pu)"; Tf "WOF time constant (s)"
      mask init: same as VFlexP/Grid/DCAC converters/DC_VCVSC/VI
  vidref : Outport
  viqref : Outport  Port=2
  wires:
  Product/1 -> Sum8/1
  Sum14/1 -> PIvd/1(ref)  "vodref"
  RC/2(vq) -> [voq], viqref/1, RL/4(v_out_q), Sum6/2, PIvq/2(y), Cf/1, Real-Imag to Complex4/2  "voq"
  [omega] -> Product/2
  Lf1/1 -> Product3/2
  Fi/1 -> Sum4/1
  Sum15/1 -> PIvq/1(ref)  "voqref"
  Product3/1 -> Sum9/2
  Product2/1 -> Sum3/2
  Cf 1/1 -> Product2/2
  Cf/1 -> Product1/2
  Product1/1 -> Sum2/1
  iod/1 -> RC/2(i_d_out), Real-Imag to Complex5/1, Product4/2, Fi/1  "iod"
  Sum2/1 -> Sum4/2
  "Lf "/1 -> Product/1
  Sum3/1 -> Sum5/1
  [omega] -> RC/5(omega), RL/5(omega), Product3/1  "omega"
  ioq/1 -> RC/4(i_q_out), Fi2/1, Real-Imag to Complex5/2, Product5/2  "ioq"
  Fi2/1 -> Sum5/2
  PIvd/1(Out1) -> Sum2/2
  PIvq/1(Out1) -> Sum3/1
  PIid/1(Out1) -> Sum8/2
  PIiq/1(Out1) -> Sum9/1
  omega/1 -> Product2/1, [omega]  "omega"
  [omega] -> Product1/1
  RL/1(id) -> RC/1(i_d_in), Scope2/1, Real-Imag to Complex2/1, PIid/2(y), Lf1/1
  RL/2(iq) -> Scope4/1, PIiq/2(y), "Lf "/1, Real-Imag to Complex2/2, RC/3(i_q_in)
  Sum8/1 -> Sum1/2  "vidref"
  Sum9/1 -> Sum6/1  "viqref"
  Sum1/1 -> RL/1(v_in_d)
  Sum6/1 -> RL/3(v_in_q)
  Sum4/1 -> Real-Imag to Complex3/1, [ildref]  "ildref"
  Sum5/1 -> Real-Imag to Complex3/2, [ilqref]  "ilqref"
  RC/1(vd) -> Real-Imag to Complex4/1, RL/2(v_out_d), Sum1/1, [vod], vidref/1, PIvd/2(y), Cf 1/1
  Complex to Real-Imag1/2 -> Scope4/2, PIiq/1(ref)
  Real-Imag to Complex2/1 -> Complex to Magnitude-Angle2/1
  Complex to Magnitude-Angle2/1 -> Scope1/1  "i_mod"
  Complex to Real-Imag1/1 -> Scope2/2, PIid/1(ref)
  Real-Imag to Complex3/1 -> Complex to Magnitude-Angle3/1
  Saturation/1 -> Magnitude-Angle to Complex/1, Scope3/1, Relational Operator/1
  Relational Operator/1 -> PIvd/3(anti_windup), PIvq/3(anti_windup), NOT/1
  Complex to Magnitude-Angle3/1 -> Scope6/1, Relational Operator/2, Saturation/1
  Magnitude-Angle to Complex/1 -> Complex to Real-Imag1/1
  Complex to Magnitude-Angle3/2 -> Magnitude-Angle to Complex/2
  Complex to Magnitude-Angle4/1 -> Scope7/1  "vc_mod"
  Real-Imag to Complex4/1 -> Complex to Magnitude-Angle4/1
  Real-Imag to Complex5/1 -> Complex to Magnitude-Angle5/1
  Complex to Magnitude-Angle5/1 -> Scope8/1  "io_mod"
  vodref/1 -> Sum14/2  "vodref"
  voqref/1 -> Sum15/1  "voqref"
  NOT/1 -> Memory/1
  VI/1(vd) -> Sum14/1
  VI/2(vq) -> Sum15/2
  Memory/1 -> Product5/1, Product4/1
  Product4/1 -> VI/1(id)
  Product5/1 -> VI/2(iq)

== system VFlexP/Grid/Generators/GFr/VCC/static ==
  vodref : Inport
  voqref : Inport  Port=2
  iod : Inport  Port=3
  ioq : Inport  Port=4
  omega : Inport  Port=5
  Terminator : Terminator
  Terminator1 : Terminator
  Terminator2 : Terminator
  vidref : Outport
  viqref : Outport  Port=2
  wires:
  voqref/1 -> viqref/1  "voqref"
  vodref/1 -> vidref/1  "vodref"
  iod/1 -> Terminator/1  "iod"
  ioq/1 -> Terminator1/1  "ioq"
  omega/1 -> Terminator2/1  "ioq"

== system VFlexP/Grid/Generators/GFr/VI/WOF_d ==
  In1 : Inport
  Gain : Gain  Gain=iTf
  I : Integrator  InitialConditionSource=external  InitialCondition=Grid_op_VCVSC.op.States(16).x'
  Sum : Sum  Inputs=+-|
  Sum4 : Sum  Inputs=|+-
  Out1 : Outport
  wires:
  Sum/1 -> Out1/1
  I/1 -> Sum4/2, Sum/2
  In1/1 -> Sum4/1, Sum/1, I/2
  Sum4/1 -> Gain/1
  Gain/1 -> I/1

== system VFlexP/Grid/Generators/GFr/VI/WOF_q ==
  In1 : Inport
  Gain : Gain  Gain=iTf
  I : Integrator  InitialConditionSource=external  InitialCondition=Grid_op_VCVSC.op.States(17).x'
  Sum : Sum  Inputs=+-|
  Sum4 : Sum  Inputs=|+-
  Out1 : Outport
  wires:
  Sum/1 -> Out1/1
  I/1 -> Sum4/2, Sum/2
  In1/1 -> Sum4/1, Sum/1, I/2
  Sum4/1 -> Gain/1
  Gain/1 -> I/1

== system VFlexP/Grid/Generators/IG/PQ/LPF_P ==
  P : Inport
  Gain : Gain  Gain=100
  I : Integrator  InitialCondition=Grid_op_IG.op.States(3).x'
  Sum4 : Sum  Inputs=|+-
  P_f : Outport
  wires:
  Gain/1 -> I/1
  Sum4/1 -> Gain/1
  P/1 -> Sum4/1
  I/1 -> P_f/1, Sum4/2

== system VFlexP/Grid/Generators/IG/PQ/LPF_Q ==
  Q : Inport
  Gain : Gain  Gain=100
  I : Integrator  InitialCondition=Grid_op_IG.op.States(4).x'
  Sum4 : Sum  Inputs=|+-
  Q_f : Outport
  wires:
  Gain/1 -> I/1
  Q/1 -> Sum4/1
  I/1 -> Q_f/1, Sum4/2
  Sum4/1 -> Gain/1

== system VFlexP/Grid/Generators/IG/RL out/dynamic ==
  v_in_d : Inport
  v_out_d : Inport  Port=2
  v_in_q : Inport  Port=3
  v_out_q : Inport  Port=4
  Gain1 : Gain  Gain=L
  Gain2 : Gain  Gain=R
  Gain3 : Gain  Gain=R
  Gain4 : Gain  Gain=L
  Gain5 : Gain  Gain=invL
  Gain7 : Gain  Gain=invL
  Product{,1..3} (4 alike) : Product
  Selector1 : Selector  InputPortWidth=length(fref.ref_units)  IndexOptions=Index vector (dialog)  Indices=block_fref  OutputSizes=1
  Selector8 : Selector  InputPortWidth=length(fref.ref_units)  IndexOptions=Index vector (dialog)  Indices=block_fref  OutputSizes=1
  Sum4 : Sum  Inputs=+-|
  Sum5 : Sum  Inputs=|-+
  Sum6 : Sum  Inputs=|++
  Sum7 : Sum  Inputs=-+|
  Sum8 : Sum  Inputs=|+-
  Sum9 : Sum  Inputs=-+|
  i_d : Integrator  InitialCondition=Grid_op_IG.op.States(5).x'
  i_q : Integrator  InitialCondition=Grid_op_IG.op.States(6).x'
  id : Outport
  iq : Outport  Port=2
  v_outd : Outport  Port=3
  v_outq : Outport  Port=4
  wires:
  v_out_q/1 -> v_outq/1, Sum9/1  "v_out_q"
  v_out_d/1 -> v_outd/1, Sum7/1  "v_out_d"
  Sum9/1 -> Sum8/1
  Gain1/1 -> Product1/2
  i_q/1 -> iq/1, Gain4/1, Gain3/1  "iq"
  Sum5/1 -> Sum9/2
  Gain3/1 -> Sum5/1
  Sum7/1 -> Sum6/1
  Gain4/1 -> Product/1
  Product1/1 -> Sum8/2
  Sum4/1 -> Sum7/2
  Sum8/1 -> Gain7/1
  Product/1 -> Sum6/2
  [omega_ref] -> Selector1/1  "omega"
  Sum6/1 -> Gain5/1
  i_d/1 -> id/1, Gain1/1, Gain2/1  "id"
  Gain2/1 -> Sum4/2
  v_in_d/1 -> Sum4/1  "v_in_d"
  v_in_q/1 -> Sum5/2  "v_in_q"
  [omega_base] -> Selector8/1
  Selector8/1 -> Product2/1, Product3/2
  Product3/1 -> i_d/1
  Product2/1 -> i_q/1
  Gain7/1 -> Product2/2
  Selector1/1 -> Product/2, Product1/1
  Gain5/1 -> Product3/1

== system VFlexP/Grid/Generators/IG/RL out/static ==
  v_in_d : Inport
  v_out_d : Inport  Port=2
  v_in_q : Inport  Port=3
  v_out_q : Inport  Port=4
  Constant : Constant  Value=R.^2
  Constant1 : Constant
  Divide : Product  Inputs=*/
  Gain : Gain  Gain=L
  Gain1 : Gain  Gain=R
  Gain2 : Gain  Gain=R
  Product{,1..5} (6 alike) : Product
  Selector8 : Selector  InputPortWidth=length(fref.ref_units)  IndexOptions=Index vector (dialog)  Indices=block_fref  OutputSizes=1
  Sum : Sum  Inputs=|++
  Sum1 : Sum  Inputs=|+-
  Sum2 : Sum  Inputs=|+-
  Sum3 : Sum  Inputs=|++
  Sum4 : Sum  Inputs=|-+
  id : Outport
  iq : Outport  Port=2
  v_outd : Outport  Port=3
  v_outq : Outport  Port=4
  wires:
  [omega_ref] -> Selector8/1  "omega"
  v_in_d/1 -> Sum1/1  "v_in_d"
  v_out_q/1 -> v_outq/1, Sum2/2  "v_out_q"
  Sum4/1 -> iq/1  "iq"
  Sum3/1 -> id/1  "id"
  Gain1/1 -> Product1/2
  Product2/1 -> Product4/2, Product3/1
  Product4/1 -> Sum4/1
  Divide/1 -> Gain2/1, Gain1/1, Product2/1
  Sum1/1 -> Product1/1, Product4/1  "vd"
  Product3/1 -> Sum3/2
  Constant1/1 -> Divide/1
  Gain/1 -> Product/2, Product/1, Product2/2
  Sum2/1 -> Product5/1, Product3/2  "vq"
  Constant/1 -> Sum/1
  Product5/1 -> Sum4/2
  Product1/1 -> Sum3/1
  Product/1 -> Sum/2
  Gain2/1 -> Product5/2
  Sum/1 -> Divide/2
  v_out_d/1 -> v_outd/1, Sum1/2  "v_out_d"
  v_in_q/1 -> Sum2/1  "v_in_q"
  Selector8/1 -> Gain/1

== system VFlexP/Grid/Generators/IG/RL out/static_omega ==
  v_in_d : Inport
  v_out_d : Inport  Port=2
  v_in_q : Inport  Port=3
  v_out_q : Inport  Port=4
  Gain : Gain  Gain=1./(R.^2+L.^2)
  Gain2 : Gain  Gain=1./(R.^2+L.^2)
  Gain3 : Gain  Gain=R
  Gain4 : Gain  Gain=L
  Gain5 : Gain  Gain=L
  Gain6 : Gain  Gain=R
  Sum : Sum  Inputs=|++
  Sum1 : Sum  Inputs=|+-
  Sum2 : Sum  Inputs=|+-
  Sum3 : Sum  Inputs=|-+
  id : Outport
  iq : Outport  Port=2
  v_outd : Outport  Port=3
  v_outq : Outport  Port=4
  wires:
  v_in_q/1 -> Sum2/1  "v_in_q"
  v_in_d/1 -> Sum1/1  "v_in_d"
  v_out_q/1 -> v_outq/1, Sum2/2  "v_out_q"
  v_out_d/1 -> v_outd/1, Sum1/2  "v_out_d"
  Sum1/1 -> Gain/1  "vd"
  Sum2/1 -> Gain2/1  "vq"
  Gain/1 -> Gain5/1, Gain3/1
  Gain3/1 -> Sum/1
  Gain4/1 -> Sum/2
  Gain2/1 -> Gain6/1, Gain4/1
  Sum/1 -> id/1
  Gain5/1 -> Sum3/1
  Sum3/1 -> iq/1
  Gain6/1 -> Sum3/2

== system VFlexP/Grid/Generators/MGES/Electromagnetic/order 2 ==
  vsd : Inport
  vsq : Inport  Port=2
  ws : Inport  Port=3
  Gain : Gain  Gain=1./Lssd_pu
  Gain1 : Gain  Gain=Rs_pu
  Gain17 : Gain  Gain=-1
  Gain2 : Gain  Gain=Rs_pu
  Gain3 : Gain  Gain=1./Lssd_pu
  Gain4 : Gain
  Gain5 : Gain
  Gain6 : Gain  Gain=-1
  Gain7 : Gain  Gain=-1
  Integrator : Integrator  InitialCondition=Grid_op_MGES.op.States(5).x'
  Matrix Concatenate : Concatenate  Mode=Multidimensional array
  Product{1..4} (4 alike) : Product
  Scope : Scope  NumInputPorts=2
      settings: ActiveDisplayYMinimum=-176.647  ActiveDisplayYMaximum=19.6557
  Selector2 : Selector  InputPortWidth=length(fref.ref_units)  IndexOptions=Index vector (dialog)  Indices=block_fref  OutputSizes=1
  Sum : Sum  Inputs=|++
  Sum1 : Sum  Inputs=-|+|-  InputSameDT=on  SaturateOnIntegerOverflow=on  OutDataTypeStr=Inherit: Same as first input
  Sum2 : Sum  Inputs=-|+|-  InputSameDT=on  SaturateOnIntegerOverflow=on  OutDataTypeStr=Inherit: Same as first input
  psis_d : Integrator  InitialCondition=Grid_op_MGES.op.States(6).x'
  psis_q : Integrator  InitialCondition=Grid_op_MGES.op.States(7).x'
  isd : Outport  VectorParamsAs1DForOutWhenUnconnected=off
  isq : Outport  Port=2  VectorParamsAs1DForOutWhenUnconnected=off
  psi : Outport  Port=3  VectorParamsAs1DForOutWhenUnconnected=off
  wires:
  Product4/1 -> Scope/1, psis_d/1
  vsd/1 -> Sum2/2
  ws/1 -> Product1/1, Product2/2
  Matrix Concatenate/1 -> psi/1
  Product3/1 -> psis_q/1
  Sum1/1 -> Product3/1
  Product1/1 -> Sum2/1
  Product2/1 -> Sum1/3
  Sum2/1 -> Product4/2
  psis_q/1 -> Sum/1, Matrix Concatenate/2, Gain17/1  "psis_q"
  Gain1/1 -> Sum1/1
  [omega_base] -> Selector2/1
  vsq/1 -> Sum1/2
  Gain/1 -> Gain4/1, Gain6/1
  Gain2/1 -> Sum2/3
  Gain3/1 -> Gain5/1, Gain7/1
  Gain17/1 -> Product1/2
  Selector2/1 -> Product4/1, Product3/2
  Sum/1 -> Gain3/1
  Integrator/1 -> Sum/2
  Gain4/1 -> Gain2/1
  Gain5/1 -> Gain1/1
  psis_d/1 -> Product2/1, Matrix Concatenate/1, Gain/1, Scope/2
  Gain6/1 -> isd/1
  Gain7/1 -> isq/1

== system VFlexP/Grid/Generators/MGES/Electromagnetic/order 8 ==
  vsd : Inport
  vsq : Inport  Port=2
  vfd : Inport  Port=3
  ws : Inport  Port=4
  Stator circuit : Subsystem
  psi->i : Subsystem
  isd : Outport
  isq : Outport  Port=2
  psi : Outport  Port=3
  ifd : Outport  Port=4
  wires:
  psi->i/3(isq) -> isq/1
  psi->i/2(i) -> Stator circuit/3(i)
  vsd/1 -> Stator circuit/1(vsd)
  vsq/1 -> Stator circuit/2(vsq)
  ws/1 -> Stator circuit/4(ws)
  Stator circuit/1(psi) -> psi/1, psi->i/1(psi)
  vfd/1 -> Stator circuit/5(vfd)
  psi->i/1(isd) -> isd/1
  psi->i/4(ifd) -> ifd/1

== system VFlexP/Grid/Generators/MGES/Electromagnetic/order 8 nomatrix ==
  vsd : Inport
  vsq : Inport  Port=2
  vfd : Inport  Port=3
  ws : Inport  Port=4
  Assignment : Assignment  NumberOfDimensions=2  DiagnosticForDimensions=Warning  IndexOptions=Index vector (dialog),Assign all  Indices=2,1  OutputSizes=1,1
  Constant : Constant  Value=Lfd_pu  VectorParams1D=off
  Integrator : Integrator  InitialCondition=Grid_op_MGES.op.States(5).x'
  Selector : Selector  NumberOfDimensions=2  InputPortWidth=3  IndexOptions=Index vector (dialog),Select all  Indices=2,1  OutputSizes=1,1
  Stator circuit : Subsystem
  Sum3 : Sum  Inputs=++|
  Switch6 : Switch  Criteria=u2 ~= 0  SaturateOnIntegerOverflow=off  InputSameDT=off
  psi->i : Subsystem
  isd : Outport
  isq : Outport  Port=2
  psi : Outport  Port=3
  wires:
  psi->i/3(isq) -> isq/1
  psi->i/2(i) -> Stator circuit/3(i)
  vsd/1 -> Stator circuit/1(vsd)
  vsq/1 -> Stator circuit/2(vsq)
  ws/1 -> Stator circuit/4(ws)
  Stator circuit/1(psi) -> psi/1, Selector/1, Assignment/1
  vfd/1 -> Stator circuit/5(vfd)
  psi->i/1(isd) -> isd/1
  Sum3/1 -> Switch6/3
  Constant/1 -> Switch6/2
  Integrator/1 -> Sum3/2
  Assignment/1 -> psi->i/1(psi)
  Selector/1 -> Sum3/1, Switch6/1
  Switch6/1 -> Assignment/2

== system VFlexP/Grid/Generators/MGES/LeadLag/AVR_LeadLag ==
  In1 : Inport
  Gain : Gain  Gain=1./T_1
  Gain2 : Gain  Gain=T_2./T_1
  Sum : Sum  Inputs=|+-
  Sum1 : Sum  Inputs=++|
  x_f : Integrator  InitialConditionSource=external  InitialCondition=Grid_op_MGES.op.States(20).x'
  Out1 : Outport
  wires:
  x_f/1 -> Sum1/2, Sum/2
  Gain/1 -> x_f/1
  Sum/1 -> Gain/1, Gain2/1
  Gain2/1 -> Sum1/1
  Sum1/1 -> Out1/1
  In1/1 -> x_f/2, Sum/1

== system VFlexP/Grid/Generators/MGES/Subsystem/LPF1 ==
  in : Inport
  Gain : Gain  Gain=1./T_s
  Sum4 : Sum  Inputs=|+-
  x_a : Integrator  InitialConditionSource=external  InitialCondition=Grid_op_MGES.op.States(26).x'
  out : Outport
  wires:
  x_a/1 -> Sum4/2, out/1
  in/1 -> x_a/2, Sum4/1
  Sum4/1 -> Gain/1
  Gain/1 -> x_a/1

== system VFlexP/Grid/Generators/MGES/Subsystem/LPF2 ==
  in : Inport
  Gain : Gain  Gain=1./T_s
  Sum4 : Sum  Inputs=|+-
  x_a : Integrator  InitialConditionSource=external  InitialCondition=Grid_op_MGES.op.States(27).x'
  out : Outport
  wires:
  x_a/1 -> Sum4/2, out/1
  in/1 -> x_a/2, Sum4/1
  Sum4/1 -> Gain/1
  Gain/1 -> x_a/1

== system VFlexP/Grid/Generators/MGES/Subsystem/LPF3 ==
  in : Inport
  Gain : Gain  Gain=1./T_s
  Sum4 : Sum  Inputs=|+-
  x_a : Integrator  InitialConditionSource=external  InitialCondition=Grid_op_MGES.op.States(28).x'
  out : Outport
  wires:
  x_a/1 -> Sum4/2, out/1
  in/1 -> x_a/2, Sum4/1
  Sum4/1 -> Gain/1
  Gain/1 -> x_a/1

== system VFlexP/Grid/Generators/MGES/Subsystem/LPF4 ==
  in : Inport
  Gain : Gain  Gain=1./T_s
  Sum4 : Sum  Inputs=|+-
  x_a : Integrator  InitialConditionSource=external  InitialCondition=Grid_op_MGES.op.States(29).x'
  out : Outport
  wires:
  x_a/1 -> Sum4/2, out/1
  in/1 -> x_a/2, Sum4/1
  Sum4/1 -> Gain/1
  Gain/1 -> x_a/1

== system VFlexP/Grid/Generators/MGES/Subsystem/LPF7 ==
  in : Inport
  Gain : Gain  Gain=1./T_s
  Sum4 : Sum  Inputs=|+-
  x_a : Integrator  InitialConditionSource=external  InitialCondition=Grid_op_MGES.op.States(30).x'
  out : Outport
  wires:
  x_a/1 -> Sum4/2, out/1
  in/1 -> x_a/2, Sum4/1
  Sum4/1 -> Gain/1
  Gain/1 -> x_a/1

== system VFlexP/Grid/Generators/MSG/GRID CONVERTER CONTROL/PI Estator Current d ==
  in : Inport
  Gain : Gain  Gain=Kp_ia
  Gain1 : Gain  Gain=Ki_ia
  Sum : Sum  Inputs=++|
  xa2 : Integrator  InitialCondition=Grid_op_MSG.op.States(1).x'
  out : Outport  VectorParamsAs1DForOutWhenUnconnected=off
  wires:
  xa2/1 -> Sum/2
  Gain/1 -> Sum/1
  in/1 -> Gain1/1, Gain/1
  Sum/1 -> out/1
  Gain1/1 -> xa2/1

== system VFlexP/Grid/Generators/MSG/GRID CONVERTER CONTROL/PI Estator Current q ==
  in : Inport
  Gain : Gain  Gain=Kp_ia
  Gain1 : Gain  Gain=Ki_ia
  Sum : Sum  Inputs=++|
  xa1 : Integrator  InitialCondition=Grid_op_MSG.op.States(2).x'
  out : Outport  VectorParamsAs1DForOutWhenUnconnected=off
  wires:
  Gain1/1 -> xa1/1
  Sum/1 -> out/1
  in/1 -> Gain/1, Gain1/1
  Gain/1 -> Sum/1
  xa1/1 -> Sum/2

== system VFlexP/Grid/Generators/MSG/GRID CONVERTER CONTROL/Subsystem1 ==
  ws : Inport
  vaq' : Inport  Port=2
  iad : Inport  Port=3
  Gain1 : Gain  Gain=La_pu
  Product1 : Product
  Sum4 : Sum  Inputs=-|-  InputSameDT=on  SaturateOnIntegerOverflow=on  OutDataTypeStr=Inherit: Same as first input
  vadq : Outport
  wires:
  iad/1 -> Product1/2
  Gain1/1 -> Product1/1
  vaq'/1 -> Sum4/1
  Sum4/1 -> vadq/1  "vadq"
  Product1/1 -> Sum4/2
  ws/1 -> Gain1/1

== system VFlexP/Grid/Generators/MSG/GRID CONVERTER CONTROL/Subsystem3 ==
  vad' : Inport
  vd : Inport  Port=2
  iaq : Inport  Port=3
  ws : Inport  Port=4
  Gain1 : Gain  Gain=La_pu
  Product1 : Product
  Sum4 : Sum  Inputs=-|+|+  InputSameDT=on  SaturateOnIntegerOverflow=on  OutDataTypeStr=Inherit: Same as first input
  vad : Outport
  wires:
  iaq/1 -> Product1/2
  ws/1 -> Gain1/1
  Product1/1 -> Sum4/3
  Sum4/1 -> vad/1  "vadq"
  vd/1 -> Sum4/2
  vad'/1 -> Sum4/1
  Gain1/1 -> Product1/1

== system VFlexP/Grid/Generators/MSG/MACHINE CONVERTER CONTROL/PI Estator Current d ==
  in : Inport
  Gain : Gain  Gain=Kpd_m
  Gain1 : Gain  Gain=Kid_m
  Sum : Sum  Inputs=++|
  xs1 : Integrator  InitialCondition=Grid_op_MSG.op.States(3).x'
  out : Outport  VectorParamsAs1DForOutWhenUnconnected=off
  wires:
  xs1/1 -> Sum/2
  Gain/1 -> Sum/1
  in/1 -> Gain1/1, Gain/1
  Sum/1 -> out/1
  Gain1/1 -> xs1/1

== system VFlexP/Grid/Generators/MSG/MACHINE CONVERTER CONTROL/PI Estator Current q ==
  in : Inport
  Gain : Gain  Gain=Kpq_m
  Gain1 : Gain  Gain=Kiq_m
  Sum : Sum  Inputs=++|
  xs2 : Integrator  InitialCondition=Grid_op_MSG.op.States(4).x'
  out : Outport  VectorParamsAs1DForOutWhenUnconnected=off
  wires:
  Gain1/1 -> xs2/1
  Sum/1 -> out/1
  in/1 -> Gain/1, Gain1/1
  Gain/1 -> Sum/1
  xs2/1 -> Sum/2

== system VFlexP/Grid/Generators/MSG/MACHINE CONVERTER CONTROL/Subsystem1 ==
  wr : Inport
  vsq' : Inport  Port=2
  isd : Inport  Port=3
  ifd : Inport  Port=4
  Constant : Constant  Value=Lssd_pu
  Constant1 : Constant  Value=Lmd_pu
  Product1 : Product
  Product2 : Product
  Product3 : Product
  Sum : Sum
  Sum4 : Sum  InputSameDT=on  SaturateOnIntegerOverflow=on  OutDataTypeStr=Inherit: Same as first input
  vsq : Outport
  wires:
  isd/1 -> Product1/2
  Constant/1 -> Product1/1
  vsq'/1 -> Sum4/1
  Sum4/1 -> vsq/1  "vsq"
  Constant1/1 -> Product2/1
  ifd/1 -> Product2/2
  Product1/1 -> Sum/1
  Product2/1 -> Sum/2
  wr/1 -> Product3/2
  Sum/1 -> Product3/1
  Product3/1 -> Sum4/2

== system VFlexP/Grid/Generators/MSG/MACHINE CONVERTER CONTROL/Subsystem3 ==
  vsd' : Inport
  isq : Inport  Port=2
  wr : Inport  Port=3
  Gain1 : Gain  Gain=Lssq_pu
  Product1 : Product
  Sum4 : Sum  Inputs=+|-  InputSameDT=on  SaturateOnIntegerOverflow=on  OutDataTypeStr=Inherit: Same as first input
  vsd : Outport
  wires:
  isq/1 -> Product1/2
  wr/1 -> Gain1/1
  Product1/1 -> Sum4/2
  Sum4/1 -> vsd/1  "vsd"
  vsd'/1 -> Sum4/1
  Gain1/1 -> Product1/1
